simulink model "W_integ_ClientServer_Model"  (R2024b)
settings: Solver=FixedStepDiscrete  StartTime=0.0  StopTime=10.0  FixedStep=0.05  RelTol=1e-3
undefined symbols (not defined in the file or in its folder): call_ServerService_getDataC, call_ServerService_setDataA, call_ServerService_setDataB
settings Model: Tag=EP_AA_WRAPPER_INTEGRATION  DataDictionary=Wrapper_ClientServer_Model.sldd  Creator=yatishc  LastModifiedBy=nabilekhoury
settings OptimizationCC: DefaultParameterBehavior=Inlined  EnhancedBackFolding=on  PassReuseOutputArgsAs=Individual arguments  ZeroExternalMemoryAtStartup=off  ZeroInternalMemoryAtStartup=off  OptimizeBlockOrder=speed  DifferentSizesBufferReuse=on  OptimizationCustomize=off  EfficientTunableParamExpr=on
settings DebuggingCC: ParameterTunabilityLossMsg=error
settings ModelReferenceCC: ModelReferenceNumInstancesAllowed=Single
settings SFSimCC: SimGenImportedTypeDefs=on  MATLABDynamicMemAlloc=off  SimTargetLang=C++
settings RTWCC: Description=Embedded Coder  SystemTargetFile=ert.tlc  GenCodeOnly=on  TemplateMakefile=ert_default_tmf  CustomSourceCode="#include \"ClientServer_Model_adapter.h\""  CustomInitializer=sut_initialize();  DataTypeReplacement=CDataTypesFixedWidth  TargetLang=C++
settings CodeAppCC: ForceParamTrailComments=on  IgnoreCustomStorageClasses=off  MaxIdLength=256  OperatorAnnotations=on  SimulinkDataObjDesc=on  SFDataObjDesc=on  CustomSymbolStrGlobalVar=w_$R$N$M  CustomSymbolStrType=w_$N$R$M_T  InsertBlockDesc=on
settings ERTTargetCC: TargetLangStandard=C++17 (ISO)  GenerateSampleERTMain=on  ERTCustomFileTemplate=example_file_process.tlc  MaxIdInt64=INT64_MAX  MinIdInt64=INT64_MIN  MaxIdUint64=UINT64_MAX  MaxIdInt32=INT32_MAX  MinIdInt32=INT32_MIN  MaxIdUint32=UINT32_MAX  MaxIdInt16=INT16_MAX  MinIdInt16=INT16_MIN  MaxIdUint16=UINT16_MAX  MaxIdInt8=INT8_MAX  MinIdInt8=INT8_MIN  MaxIdUint8=UINT8_MAX

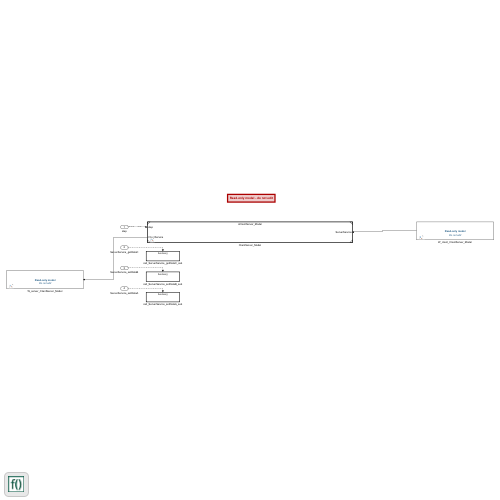
[thumbnail: Simulink's stored preview of the top-level diagram]
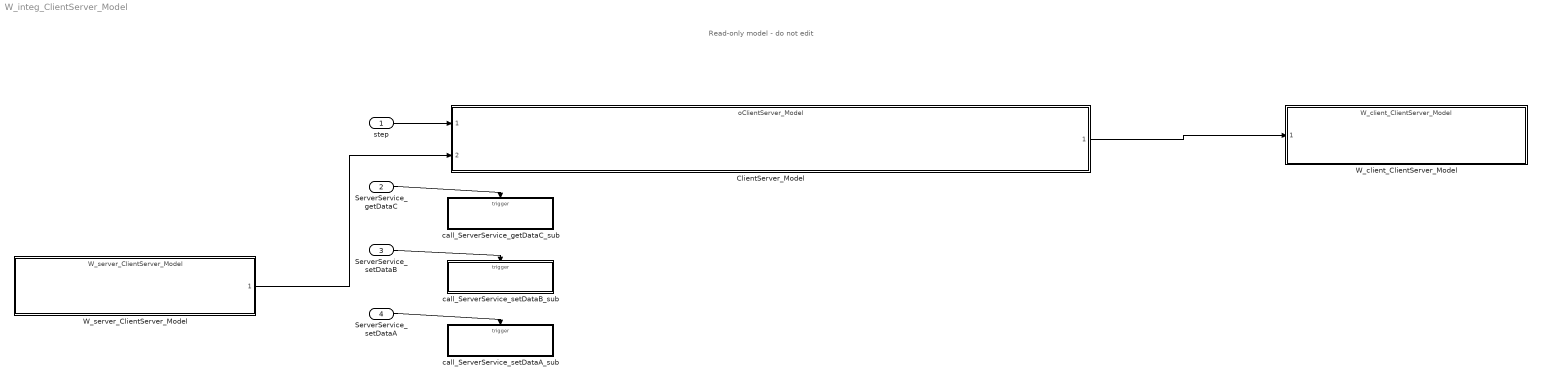
== system W_integ_ClientServer_Model ==
  note: Read-only model - do not edit
  step : Inport  PortDimensions=1  OutputFunctionCall=on
  ServerService_getDataC : Inport  Port=2  OutputFunctionCall=on
  ServerService_setDataB : Inport  Port=3  OutputFunctionCall=on
  ServerService_setDataA : Inport  Port=4  OutputFunctionCall=on
  ClientServer_Model : ModelReference  Tag=BTC AUTOSAR Main Model Reference Block  ModelNameDialog=oClientServer_Model.slx  SimulationMode=Normal  ScheduleRates=on  ModelReferenceVersion=1.12
  W_client_ClientServer_Model : ModelReference  ModelNameDialog=W_client_ClientServer_Model  SimulationMode=Normal  ScheduleRates=on  ModelReferenceVersion=1.1
      settings: OpenFcn=open_system(gcb, 'mask');
      mask DialogControl DescGroupVar Prompt: BTC Embedded Systems mocking block
      mask DialogControl DescTextVar Prompt: This is a BTC Embedded Systems mocking block. Do not edit its contents.
      mask Display: disp('\color[rgb]{0.11,0.34,0.51}\bf Read-only model', 'texmode', 'on');disp('\color[rgb]{0.11,0.34,0.51}\newline\newline\rm\it Do not edit', 'texmode', 'on');
  W_server_ClientServer_Model : ModelReference  ModelNameDialog=W_server_ClientServer_Model  SimulationMode=Normal  ScheduleRates=on  ModelReferenceVersion=1.1
      settings: OpenFcn=open_system(gcb, 'mask');
      mask DialogControl DescGroupVar Prompt: BTC Embedded Systems mocking block
      mask DialogControl DescTextVar Prompt: This is a BTC Embedded Systems mocking block. Do not edit its contents.
      mask Display: disp('\color[rgb]{0.11,0.34,0.51}\bf Read-only model', 'texmode', 'on');disp('\color[rgb]{0.11,0.34,0.51}\newline\newline\rm\it Do not edit', 'texmode', 'on');
  call_ServerService_getDataC_sub : Subsystem  TreatAsAtomicUnit=on
  call_ServerService_setDataA_sub : Subsystem  TreatAsAtomicUnit=on
  call_ServerService_setDataB_sub : Subsystem  TreatAsAtomicUnit=on
  wires:
  step/1 -> ClientServer_Model/1
  W_server_ClientServer_Model/1 -> ClientServer_Model/2
  ClientServer_Model/1 -> W_client_ClientServer_Model/1
  ServerService_getDataC/1 -> call_ServerService_getDataC_sub/Trigger
  ServerService_setDataB/1 -> call_ServerService_setDataB_sub/Trigger
  ServerService_setDataA/1 -> call_ServerService_setDataA_sub/Trigger

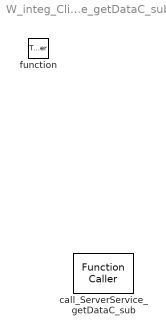
== system W_integ_ClientServer_Model/call_ServerService_getDataC_sub ==
  function : TriggerPort  TriggerType=function-call  VariantControl=(inherit)
  call_ServerService_getDataC_sub : FunctionCaller  FunctionPrototype=call_ServerService_getDataC()  InputArgumentSpecifications=<Enter example>  OutputArgumentSpecifications=<Enter example>

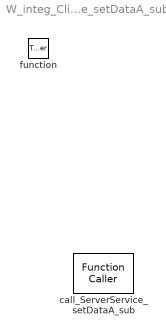
== system W_integ_ClientServer_Model/call_ServerService_setDataA_sub ==
  function : TriggerPort  TriggerType=function-call  VariantControl=(inherit)
  call_ServerService_setDataA_sub : FunctionCaller  FunctionPrototype=call_ServerService_setDataA()  InputArgumentSpecifications=<Enter example>  OutputArgumentSpecifications=<Enter example>

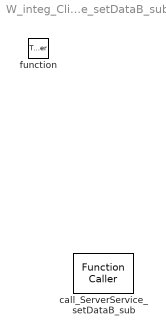
== system W_integ_ClientServer_Model/call_ServerService_setDataB_sub ==
  function : TriggerPort  TriggerType=function-call  VariantControl=(inherit)
  call_ServerService_setDataB_sub : FunctionCaller  FunctionPrototype=call_ServerService_setDataB()  InputArgumentSpecifications=<Enter example>  OutputArgumentSpecifications=<Enter example>
